simulink model "MPCModel"  (R2025b)
settings: Solver=FixedStepAuto  StartTime=0.0  StopTime=5  FixedStep=1e-6  MaxStep=1e-3  MinStep=1e-8  RelTol=1e-4
values from neighbouring files (symbols this model uses):
  cb = 0.5    [MPCVariables.mat]    (also in SkyGroundSMCVariables.mat)
  cc = 370    [MPCVariables.mat]    (also in SkyGroundSMCVariables.mat)
  Er = 12    [MPCVariables.mat]    (also in SkyGroundSMCVariables.mat)
  kb = 0.2    [MPCVariables.mat]    (also in SkyGroundSMCVariables.mat)
  ke = 62.6    [MPCVariables.mat]    (also in SkyGroundSMCVariables.mat)
  ki = 77.9    [MPCVariables.mat]    (also in SkyGroundSMCVariables.mat)
  ks = 5495    [MPCVariables.mat]    (also in SkyGroundSMCVariables.mat)
  kt = 48000    [MPCVariables.mat]    (also in SkyGroundSMCVariables.mat)
  L = 0.0128    [MPCVariables.mat]    (also in SkyGroundSMCVariables.mat)
  L_DC = 0    [MPCVariables.mat]    (also in SkyGroundSMCVariables.mat)
  ms = 82    [MPCVariables.mat]    (also in SkyGroundSMCVariables.mat)
  mu = 11.5    [MPCVariables.mat]    (also in SkyGroundSMCVariables.mat)
  R = 10.2    [MPCVariables.mat]    (also in SkyGroundSMCVariables.mat)
  Rv = 0    [MPCVariables.mat]    (also in SkyGroundSMCVariables.mat)
  vd = 0.191693290735    [MPCVariables.mat]    (also in SkyGroundSMCVariables.mat)
libraries: simulink x2, mpclib x1
settings Model: SimulationMode=accelerator  Creator=khalid  LastModifiedBy=khalid
settings SolverCC: InitialStep=1e-5  ZeroCrossAlgorithm=Adaptive
settings DataIOCC: SaveTime=off
settings DebuggingCC: MaskedZcDiagnostic=none  IgnoredZcDiagnostic=none

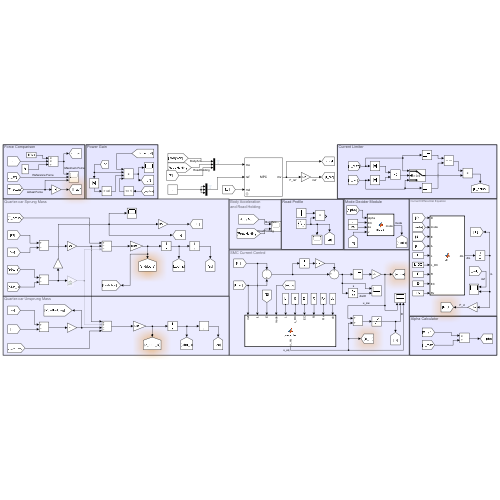
[thumbnail: Simulink's stored preview of the top-level diagram]
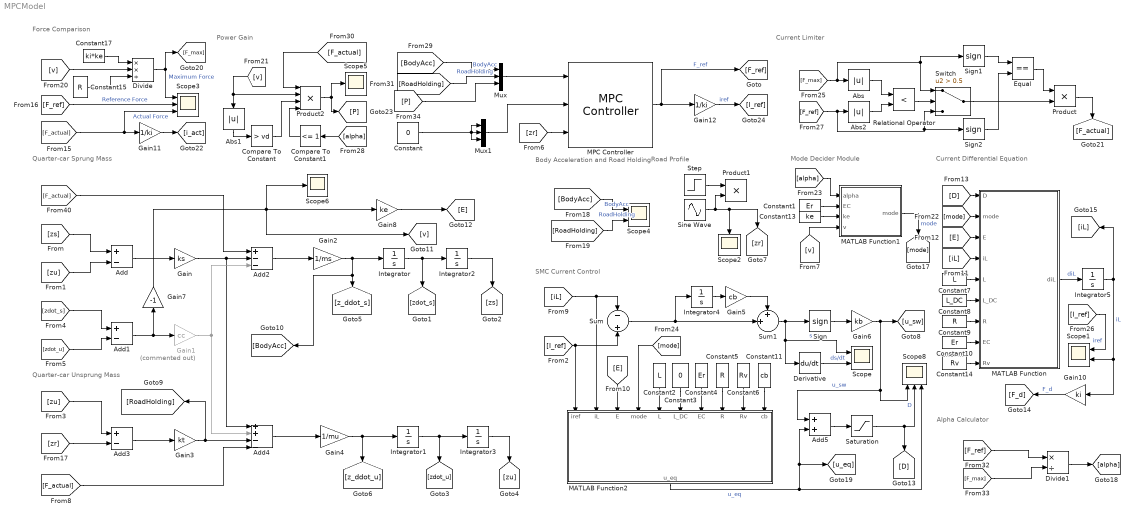
== system MPCModel ==
  note: Power Gain
  note: Road Profile
  note: Current Limiter
  note: Body Acceleration
      | and Road Holding
  note: Force Comparison
  note: Alpha Calculator
  note: Mode Decider Module
  note: Current Differential Equation
  note: SMC Current Control
  note: Quarter-car Sprung Mass
  note: Quarter-car Unsprung Mass
  Abs : Abs  SaturateOnIntegerOverflow=off
  Abs1 : Abs  SaturateOnIntegerOverflow=off
  Abs2 : Abs  SaturateOnIntegerOverflow=off
  Add : Sum  Inputs=+-
  Add1 : Sum  Inputs=+-
  Add2 : Sum  Inputs=+--
  Add3 : Sum  Inputs=+-
  Add4 : Sum  Inputs=++--
  Add5 : Sum
  Compare To Constant : simulink/Logic and Bit Operations/Compare To Constant  relop=>  const=vd  OutDataTypeStr=uint8
  Compare To Constant1 : simulink/Logic and Bit Operations/Compare To Constant  relop=<=  const=1  OutDataTypeStr=uint8
  Constant : Constant  Value=0
  Constant1 : Constant  Value=Er
  Constant10 : Constant  Value=Er
  Constant11 : Constant  Value=cb
  Constant13 : Constant  Value=ke
  Constant14 : Constant  Value=Rv
  Constant15 : Constant  Value=R
  Constant17 : Constant  Value=ki*ke
  Constant2 : Constant  Value=L
  Constant3 : Constant  Value=0
  Constant4 : Constant  Value=Er
  Constant5 : Constant  Value=R
  Constant6 : Constant  Value=Rv
  Constant7 : Constant  Value=L
  Constant8 : Constant  Value=L_DC
  Constant9 : Constant  Value=R
  Derivative : Derivative
  Divide : Product  Inputs=**/
  Divide1 : Product  Inputs=*/
  Equal : RelationalOperator  Operator===  OutDataTypeStr=boolean  RndMeth=Simplest  InputSameDT=off
  Gain : Gain  Gain=ks
  Gain1 : Gain  Commented=on  Gain=cc
  Gain10 : Gain  Gain=ki
  Gain11 : Gain  Gain=1/ki
  Gain12 : Gain  Gain=1/ki
  Gain2 : Gain  Gain=1/ms
  Gain3 : Gain  Gain=kt
  Gain4 : Gain  Gain=1/mu
  Gain5 : Gain  Gain=cb
  Gain6 : Gain  Gain=kb
  Gain7 : Gain  Gain=-1
  Gain8 : Gain  Gain=ke
  Integrator{,1..5} (6 alike) : Integrator
  MATLAB Function : MATLAB Function  TreatAsAtomicUnit=on
  MATLAB Function1 : MATLAB Function  TreatAsAtomicUnit=on
  MATLAB Function2 : MATLAB Function  TreatAsAtomicUnit=on
  MPC Controller : mpclib/MPC Controller  SCDEnableBlockLinearizationSpecification=on  is_multiple=0  enable_value=0  return_u0=off  updateMPCinCallerWorkspace=on  md_inport=on  mv_inport=off  uref_inport=off  return_cost=off  return_mvseq=off  return_qpstatus=off  return_xseq=off  return_state=off  return_ovseq=off  state_inport=off  umin_inport=off  umax_inport=off  ymin_inport=off  ymax_inport=off  cc_inport=off  ywt_inport=off  uwt_inport=off  duwt_inport=off  rhoeps_inport=off  pm_inport=off  MaximumP=10  HorizonChoice=FixedHorizon  n_ts=0.0001  n_p=10  n_mv=1  n_md=1  n_ud=0  n_mo=3  n_uo=0  BlockDataType=double  SampleTimeInherited=off  switch_inport=off
  Mux : Mux  Inputs=3
  Mux1 : Mux  Inputs=3
  Product : Product
  Product1 : Product
  Product2 : Product  Inputs=4
  Relational Operator : RelationalOperator  Operator=<  OutDataTypeStr=boolean  RndMeth=Simplest  InputSameDT=off
  Saturation : Saturate  UpperLimit=1  LowerLimit=0
  Scope : Scope  NumInputPorts=2
      settings: ActiveDisplayYMinimum=-0.72861964969167214  ActiveDisplayYMaximum=3.0272434295858131  DataLoggingVariableName=ScopeData2
  Scope1 : Scope  NumInputPorts=2
      settings: ActiveDisplayYMinimum=-1  ActiveDisplayYMaximum=1
  Scope2 : Scope
      settings: ActiveDisplayYMinimum=-0.03749999999999333  ActiveDisplayYMaximum=0.037499999999999263
  Scope3 : Scope  NumInputPorts=3
      settings: ActiveDisplayYMinimum=-367.73932008103174  ActiveDisplayYMaximum=367.04897805021483  DataLoggingVariableName=ScopeData4
  Scope4 : Scope  NumInputPorts=2
      settings: ActiveDisplayYMinimum=-4.58215637970691  ActiveDisplayYMaximum=4.5821052090116083  DataLoggingVariableName=ScopeData5
  Scope5 : Scope
      settings: ActiveDisplayYMinimum=46.701417317364843  ActiveDisplayYMaximum=54.215052566851504  DataLoggingVariableName=ScopeData3
  Scope6 : Scope
      settings: ActiveDisplayYMinimum=-0.50380828299864544  ActiveDisplayYMaximum=0.50380784340428209  DataLoggingVariableName=ScopeData6
  Scope8 : Scope  NumInputPorts=3
      settings: ActiveDisplayYMinimum=-1.7651094697775311  ActiveDisplayYMaximum=2.8491770678518753  DataLoggingVariableName=ScopeData8
  Sign : Signum
  Sign1 : Signum
  Sign2 : Signum
  Sine Wave : Sin  Amplitude=0.03  Frequency=2*pi*1.3  SampleTime=0
  Step : Step  Before=1  After=0  SampleTime=0
  Sum : Sum  Inputs=-+
  Sum1 : Sum  Inputs=+|+||
  Switch : Switch  Criteria=u2 > Threshold  Threshold=0.5  SaturateOnIntegerOverflow=off  InputSameDT=off
  wires:
  [zdot_u] -> Add1/2
  Add3/1 -> Gain3/1
  Gain3/1 -> [RoadHolding], Add4/3
  [zs] -> Add/1
  Add1/1 -> Gain1/1, Gain7/1
  [zr] -> Add3/2
  Add4/1 -> Gain4/1
  Integrator/1 -> Integrator2/1, [zdot_s]
  [zu] -> Add/2
  [F_actual] -> Add4/4
  [zdot_s] -> Add1/1
  Gain2/1 -> Integrator/1, [BodyAcc], [z_ddot_s]
  Gain/1 -> Add4/1, Add2/2
  Add/1 -> Gain/1
  Gain4/1 -> Integrator1/1, [z_ddot_u]
  [zu] -> Add3/1
  Add2/1 -> Gain2/1
  Integrator3/1 -> [zu]
  Integrator1/1 -> Integrator3/1, [zdot_u]
  Integrator2/1 -> [zs]
  [F_actual] -> Add2/1
  [BodyAcc] -> Scope4/1  "BodyAcc"
  [RoadHolding] -> Scope4/2  "RoadHolding"
  [F_actual] -> Gain11/1, Scope3/3  "Actual Force"
  Divide/1 -> [F_max], Scope3/1  "Maximum Force"
  [F_ref] -> Scope3/2  "Reference Force"
  Constant15/1 -> Divide/3
  [iL] -> MATLAB Function2/2(iL), Sum/1
  Sign/1 -> Gain6/1
  Integrator4/1 -> Gain5/1
  [I_ref] -> MATLAB Function2/1(iref), Sum/2
  Sum1/1 -> Derivative/1, Scope/1, Sign/1  "s"
  Gain6/1 -> Add5/1, Scope8/1, [u_sw]  "u_sw"
  Constant5/1 -> MATLAB Function2/8(R)
  Constant11/1 -> MATLAB Function2/10(cb)
  Constant3/1 -> MATLAB Function2/6(L_DC)
  Constant4/1 -> MATLAB Function2/7(EC)
  Constant6/1 -> MATLAB Function2/9(Rv)
  Constant2/1 -> MATLAB Function2/5(L)
  Gain8/1 -> [E]
  [E] -> MATLAB Function2/3(E)
  Add5/1 -> Saturation/1
  Saturation/1 -> Scope8/2, [D]  "D"
  Constant8/1 -> MATLAB Function/6(L_DC)
  Constant9/1 -> MATLAB Function/7(R)
  Integrator5/1 -> Scope1/2, Gain10/1, [iL]  "iL"
  MATLAB Function/1(diL) -> Integrator5/1  "diL"
  Gain10/1 -> [F_d]  "F_d"
  Constant14/1 -> MATLAB Function/9(Rv)
  Constant10/1 -> MATLAB Function/8(EC)
  Constant7/1 -> MATLAB Function/5(L)
  [iL] -> MATLAB Function/4(iL)
  [E] -> MATLAB Function/3(E)
  [D] -> MATLAB Function/1(D)
  Constant13/1 -> MATLAB Function1/3(ke)
  Constant1/1 -> MATLAB Function1/2(EC)
  [v] -> MATLAB Function1/4(v)
  MATLAB Function1/1(mode) -> [mode]  "mode"
  [mode] -> MATLAB Function/2(mode)
  [alpha] -> MATLAB Function1/1(alpha)
  [mode] -> MATLAB Function2/4(mode)
  Gain5/1 -> Sum1/1
  Constant17/1 -> Divide/1
  [v] -> Divide/2
  Abs/1 -> Relational Operator/1
  [F_ref] -> Sign2/1, Switch/3, Abs2/1
  Abs2/1 -> Relational Operator/2
  Relational Operator/1 -> Switch/2
  [F_max] -> Switch/1, Sign1/1, Abs/1
  [F_ref] -> Divide1/1
  [F_max] -> Divide1/2
  Divide1/1 -> [alpha]
  Sine Wave/1 -> [zr], Scope2/1, Product1/2
  Step/1 -> Product1/1
  Gain7/1 -> Scope6/1, Gain8/1, [v]
  [v] -> Product2/2, Abs1/1
  Product2/1 -> [P], Scope5/1
  [alpha] -> Compare To Constant1/1
  Derivative/1 -> Scope/2  "ds/dt"
  [F_actual] -> Product2/1
  [I_ref] -> Scope1/1  "iref"
  Sign1/1 -> Equal/1
  Sign2/1 -> Equal/2
  Equal/1 -> Product/1
  Switch/1 -> Product/2
  Product/1 -> [F_actual]
  Sum/1 -> Integrator4/1, Sum1/2
  Gain11/1 -> [i_act]
  Gain1/1 -> Add4/2, Add2/3
  Abs1/1 -> Compare To Constant/1
  Compare To Constant1/1 -> Product2/4
  Compare To Constant/1 -> Product2/3
  MATLAB Function2/1(u_eq) -> Add5/2, [u_eq], Scope8/3  "u_eq"
  [BodyAcc] -> Mux/1  "BodyAcc"
  [RoadHolding] -> Mux/2  "RoadHolding"
  [P] -> Mux/3
  Mux/1 -> MPC Controller/1
  Mux1/1 -> MPC Controller/2
  Constant/1 -> Mux1/1, Mux1/2, Mux1/3
  MPC Controller/1 -> [F_ref], Gain12/1  "F_ref"
  Gain12/1 -> [I_ref]  "iref"
  [zr] -> MPC Controller/3

== matlab function MPCModel/MATLAB Function1 ==
  data: alpha input; EC input; ke input; v input; mode output
function mode = mode(alpha, EC, ke, v)

    % guard against alpha >= 1
    if alpha >= 1
        % semi-active not achievable
        % both VT1 and VT2 on, passive damper
        mode = 1;   % or handle separately
        return
    end

    v_alpha = EC / (ke * (1 - alpha));

    if abs(v) < v_alpha
        mode = 1;   % boost
    else
        mode = 0;   % buck
    end
end

== matlab function MPCModel/MATLAB Function ==
  data: D input; mode input; E input; iL input; diL output; L input; L_DC input; R input; EC input; Rv input
function diL = diL(D, mode, E, iL, L, L_DC, R, EC, Rv)
    LDC = L + L_DC;
    if mode == 1  % boost
        diL = -(R/LDC)*iL - ((1-D)/LDC)*EC + (1/LDC)*E;
    else          % buck
        diL  = -((D*R*L + (1-D)*(R+Rv)*LDC)/(L * LDC))*iL - (D/LDC)*EC + (D*L + (1-D)*LDC)/(L * LDC) * E;
    end
end

== matlab function MPCModel/MATLAB Function2 ==
  data: iref input; iL input; E input; mode input; u_eq output; L input; L_DC input; EC input; R input; Rv input; cb input
function u_eq = controller(iref, iL, E, mode, L, L_DC, EC, R, Rv, cb)
    LDC = L + L_DC;
    e   = iref - iL;        % current error

    if mode == 1  % boost
        numerator   = EC - E + R*iref + cb*e*LDC;
        denominator = EC;
        u_eq = numerator / denominator;

    else          % buck
        numerator   = E - (R + Rv)*iref - cb*e*L;
        denominator = (L*R*iref)/LDC - (R + Rv)*iref + ((EC - E)*L)/LDC + E;
        u_eq = numerator / denominator;
    end
end
